simulink model "DS_distrIntp_1_10_simulated axes"  (R2019a)
settings: Solver=FixedStepDiscrete  StartTime=0.0  StopTime=inf  FixedStep=Ts  RelTol=1e-3
InitFcn:
  | %% Verwende vordefinierte Setpoints (Kreis mit Z-Komponente)
  | 
  | % Config
  | numCircles = 3;
  | scale=6;
  | %Versuch symmetrische Setpunkte zu setzen
  | pointsPerCircle =scale*(4+3*numCircles)+2;
  | 
  | r = 50;
  | m_x = r;
  | m_y = r;
  | 
  | % //
  | s = linspace(0,2*pi,pointsPerCircle);
  | 
  | setPoints_x = [];
  | setPoints_y = [];
  | 
  | for ii=1:numCircles
  | 
  | setPoints_x = [setPoints_x (-cos(s(1:floor(pointsPerCircle / 2))).*r + m_x + 2*r*(ii-1))]; %#ok<AGROW>
  | setPoints_y = [setPoints_y (sin(s).*r+m_y)]; %#ok<AGROW>pointsPerCircle / 2
  | 
  | end
  | 
  | setPoints_x = [setPoints_x flip(setPoints_x(1:end))];
  | 
  | % Loeschen doppelter y-Werte (Kreisuebergang)
  | setPoints_x(pointsPerCircle .* [1:numCircles]) = [];
  | setPoints_y(pointsPerCircle .* [1:numCircles]) = [];
  | 
  | % setPoints_x= [linspace(0,setPoints_x(19),19) setPoints_x(20:end)];
  | % setPoints_y= [linspace(0,setPoints_y(19),19) setPoints_y(20:end)];
  | 
  | % Array Elemente verschieben
  | % setPoints_x = circshift(setPoints_x,-pointsPerCircle/4,2);
  | % setPoints_y = circshift(setPoints_y,-pointsPerCircle/4,2);
  | 
  | z = zeros(1,size(setPoints_x,2));
  | z_x = -5:5;
  | z_y = -z_x.^2 + 25;
  | z_idx = 90;
  | z_idx2 = 210;
  | z(z_idx:z_idx+length(z_x)-1) = z_y;
  | z(z_idx2:z_idx2+length(z_x)-1) = z_y;
  | % z = [z_y z];
  | setPoints_z = z;
  | 
  | % setPoints_x = [zeros(1,length(z_y)) setPoints_x];
  | % setPoints_y = [setPoints_y(1,1)*ones(1,length(z_y)) setPoints_y];
  | 
  | % Umrechnung der Einheiten für Demonstrator
  | % setPoints_x = setPoints_x ./ 1000;
  | % setPoints_y = setPoints_y ./ 1000;
  | % setPoints_z = setPoints_z ./ 1000;
  | 
  | 
  | %{
  | plot(setPoints_x,setPoints_y);
  | fig = figure;
  | ... (+13 lines)
StartFcn:
  | close all;
model workspace (MAT data in the model file):
  MCOS : class17 (value not decoded)
  MCOS : class17 (value not decoded)
  MCOS : class17 (value not decoded)
  MCOS : class17 (value not decoded)
  MCOS : class17 (value not decoded)
  MCOS : class17 (value not decoded)
  MCOS : class17 (value not decoded)
  MCOS : class17 (value not decoded)
  MCOS : class17 (value not decoded)
  MCOS : class17 (value not decoded)
  MCOS : class17 (value not decoded)
  MCOS : class17 (value not decoded)
  MCOS : class17 (value not decoded)
  MCOS : class17 (value not decoded)
undefined symbols (not defined in the file or in its folder): DiscIntNeverNeededParam, VelOverride
libraries: simulink x19, vrlib x5, sldrtlib x2
(part 3 of 4)

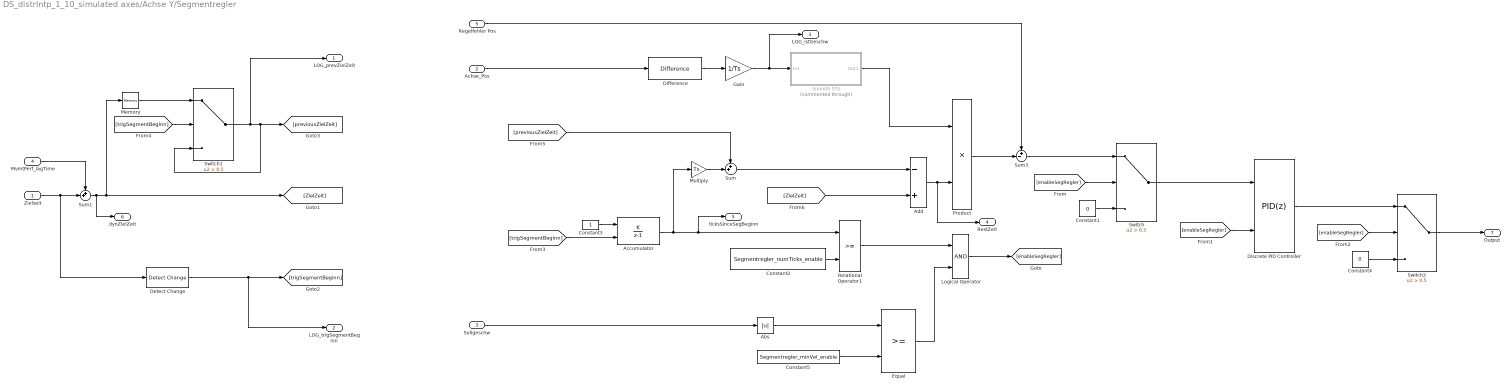
== system DS_distrIntp_1_10_simulated axes/Achse Y/Segmentregler ==
  Zielzeit : Inport
  Achse_Pos : Inport  Port=2
  Sollgeschw : Inport  Port=3
  MvmtPerf_lagTime : Inport  Port=4
  Regelfehler Pos : Inport  Port=5
  Abs : Abs
  Accumulator : DiscreteIntegrator  IntegratorMethod=Accumulation: Forward Euler  gainval=1  ExternalReset=rising  SampleTime=-1  ICPrevOutput=DiscIntNeverNeededParam  ICPrevScaledInput=DiscIntNeverNeededParam
  Add : Sum  Inputs=-+
  Constant1 : Constant  Value=0
  Constant2 : Constant  Value=Segmentregler_numTicks_enable
  Constant3 : Constant
  Constant4 : Constant  Value=0
  Constant5 : Constant  Value=Segmentregler_minVel_enable
  Detect Change : simulink/Logic and Bit Operations/Detect Change  vinit=0  OutDataTypeStr=boolean
  Difference : simulink/Discrete/Difference  ICPrevInput=0.0  OutMin=[]  OutMax=[]  OutDataType=fixdt(1, 16)  OutScaling=2^-10  DoSatur=off
  Discrete PID Controller : simulink/Continuous/PID Controller  Controller=PID  Form=Parallel  TimeDomain=Discrete-time  SampleTime=-1  IntegratorMethod=Forward Euler  FilterMethod=Forward Euler  ControllerParametersSource=internal  P=Segmentregler_P_Gain  I=Segmentregler_I_Gain  D=0  UseFilter=on  N=100  TunerSelectOption=Transfer Function Based (PID Tuner App)  InitialConditionSource=internal  InitialConditionForIntegrator=0  InitialConditionForFilter=0  DifferentiatorICPrevScaledInput=0  ExternalReset=falling  TrackingMode=off  Kt=1  LimitOutput=off  UpperSaturationLimit=inf  LowerSaturationLimit=-inf  LinearizeAsGain=off  AntiWindupMode=none  Kb=1  POutMin=[]  POutMax=[]  IOutMin=[]  IOutMax=[]  DOutMin=[]  DOutMax=[]  NOutMin=[]  NOutMax=[]  SumOutMin=[]  SumOutMax=[]  SaturationOutMin=[]  SaturationOutMax=[]  PParamMin=[]  PParamMax=[]  IParamMin=[]  IParamMax=[]  DParamMin=[]  DParamMax=[]  NParamMin=[]  NParamMax=[]  KbParamMin=[]  KbParamMax=[]  KtParamMin=[]  KtParamMax=[]  KbOutMin=[]  KbOutMax=[]  KtOutMin=[]  KtOutMax=[]  IntegratorOutMin=[]  IntegratorOutMax=[]  FilterOutMin=[]  FilterOutMax=[]  SumI1OutMin=[]  SumI1OutMax=[]  SumI2OutMin=[]  SumI2OutMax=[]  SumI3OutMin=[]  SumI3OutMax=[]  SumI4OutMin=[]  SumI4OutMax=[]  SumDOutMin=[]  SumDOutMax=[]  DifferentiatorOutMin=[]  DifferentiatorOutMax=[]  FilterDiffOutCoefMin=[]  FilterDiffOutCoefMax=[]  ReciprocalOutMin=[]  ReciprocalOutMax=[]  SumDenOutMin=[]  SumDenOutMax=[]  SumNumOutMin=[]  SumNumOutMax=[]  DivideOutMin=[]  DivideOutMax=[]  IntegratorContinuousStateAttributes=''  IntegratorStateMustResolveToSignalObject=off  IntegratorRTWStateStorageClass=Auto  FilterContinuousStateAttributes=''  FilterStateMustResolveToSignalObject=off  FilterRTWStateStorageClass=Auto  ParallelPVariant=InternalParameters  IdealPVariant=Disabled  IVariant=InternalParameters  DVariant=InternalParameters  IntegratorVariant=Discrete  SatVariant=Disabled  AWVariant=Passthrough  PCopyVariant=Disabled  TRVariant=Disabled  FdbkBlocksVariant=Forward  IdealPFdbkVariant=Disabled  SatFdbkVariant=Disabled  DerivativeFilterVariant=ForwardEulerFilter  NVariant=InternalParameters  NCopyVariant=Disabled  FilterICVariant=InternalICsFilter  IntegratorICVariant=InternalICs  ExternalResetVariant=ExternalReset  TRSumVariant=Passthrough  SumFdbkVariant=Disabled  SumVariant=Sum_PID
  Equal : RelationalOperator  OutDataTypeStr=boolean  RndMeth=Simplest
  Gain : Gain  Gain=1/Ts
  Logical Operator : Logic  AllPortsSameDT=off  OutDataTypeStr=boolean
  Memory : Memory
  Multiply : Gain  Gain=Ts
  Product : Product
  Relational Operator1 : RelationalOperator  OutDataTypeStr=boolean  RndMeth=Simplest
  Smooth 5Ts : Subsystem  Commented=through
  Sum : Sum  Inputs=++|
  Sum1 : Sum  Inputs=++|
  Sum3 : Sum  Inputs=+-|
  Switch : Switch  Criteria=u2 > Threshold  Threshold=0.5
  Switch1 : Switch  Criteria=u2 > Threshold  Threshold=0.5
  Switch2 : Switch  Criteria=u2 > Threshold  Threshold=0.5
  LOG_prevZielZeit : Outport  VectorParamsAs1DForOutWhenUnconnected=off
  LOG_trigSegmentBeginn : Outport  Port=2  VectorParamsAs1DForOutWhenUnconnected=off
  LOG_istGeschw : Outport  Port=3  VectorParamsAs1DForOutWhenUnconnected=off
  RestZeit : Outport  Port=4  VectorParamsAs1DForOutWhenUnconnected=off
  ticksSinceSegBeginn : Outport  Port=5  VectorParamsAs1DForOutWhenUnconnected=off
  dynZielZeit : Outport  Port=6  VectorParamsAs1DForOutWhenUnconnected=off
  Output : Outport  Port=7  VectorParamsAs1DForOutWhenUnconnected=off
  wires:
  MvmtPerf_lagTime/1 -> Sum1/1
  Zielzeit/1 -> Sum1/2, Detect Change/1
  Abs/1 -> Equal/1
  Sum1/1 -> [ZielZeit], Memory/1, dynZielZeit/1
  [ZielZeit] -> Add/2
  Multiply/1 -> Sum/2
  Smooth 5Ts/1(Out1) -> Product/1
  [previousZielZeit] -> Sum/1
  Switch1/1 -> [previousZielZeit], Switch1/3, LOG_prevZielZeit/1
  [trigSegmentBeginn] -> Switch1/2
  [trigSegmentBeginn] -> Accumulator/2
  Detect Change/1 -> [trigSegmentBeginn], LOG_trigSegmentBeginn/1
  Gain/1 -> Smooth 5Ts/1(In1), LOG_istGeschw/1
  Memory/1 -> Switch1/1
  Equal/1 -> Logical Operator/2
  Constant5/1 -> Equal/2
  Sollgeschw/1 -> Abs/1
  [enableSegRegler] -> Switch2/2
  [enableSegRegler] -> Discrete PID Controller/2
  [enableSegRegler] -> Switch/2
  Logical Operator/1 -> [enableSegRegler]
  Switch2/1 -> Output/1
  Regelfehler Pos/1 -> Sum3/1
  Product/1 -> Sum3/2
  Constant4/1 -> Switch2/3
  Constant1/1 -> Switch/3
  Discrete PID Controller/1 -> Switch2/1
  Achse_Pos/1 -> Difference/1
  Constant2/1 -> Relational Operator1/2
  Add/1 -> Product/2, RestZeit/1
  Relational Operator1/1 -> Logical Operator/1
  Sum/1 -> Add/1
  Switch/1 -> Discrete PID Controller/1
  Sum3/1 -> Switch/1
  Difference/1 -> Gain/1
  Accumulator/1 -> Relational Operator1/1, ticksSinceSegBeginn/1, Multiply/1
  Constant3/1 -> Accumulator/1

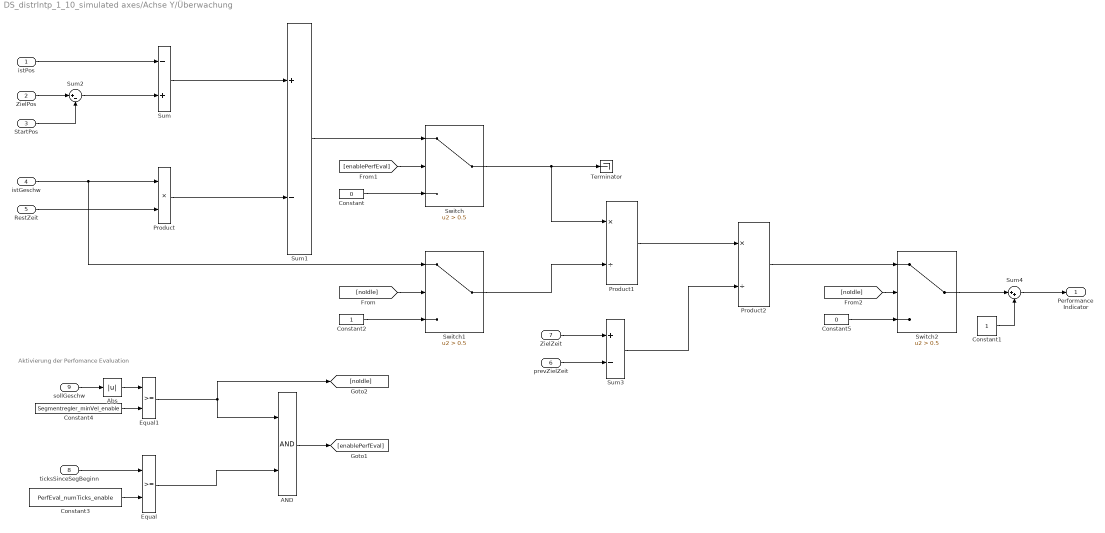
== system DS_distrIntp_1_10_simulated axes/Achse Y/Überwachung ==
  note: Aktivierung der Perfomance Evaluation
  istPos : Inport
  ZielPos : Inport  Port=2
  StartPos : Inport  Port=3
  istGeschw : Inport  Port=4
  RestZeit : Inport  Port=5
  prevZielZeit : Inport  Port=6
  ZielZeit : Inport  Port=7
  ticksSinceSegBeginn : Inport  Port=8
  sollGeschw : Inport  Port=9
  AND : Logic  AllPortsSameDT=off  OutDataTypeStr=boolean
  Abs : Abs
  Constant : Constant  Value=0
  Constant1 : Constant
  Constant2 : Constant
  Constant3 : Constant  Value=PerfEval_numTicks_enable
  Constant4 : Constant  Value=Segmentregler_minVel_enable
  Constant5 : Constant  Value=0
  Equal : RelationalOperator  OutDataTypeStr=boolean  RndMeth=Simplest
  Equal1 : RelationalOperator  OutDataTypeStr=boolean  RndMeth=Simplest
  Product : Product
  Product1 : Product  Inputs=*/
  Product2 : Product  Inputs=*/
  Sum : Sum  Inputs=-+
  Sum1 : Sum  Inputs=+-
  Sum2 : Sum  Inputs=|+-
  Sum3 : Sum  Inputs=+-
  Sum4 : Sum  Inputs=|++
  Switch : Switch  Criteria=u2 > Threshold  Threshold=0.5
  Switch1 : Switch  Criteria=u2 > Threshold  Threshold=0.5
  Switch2 : Switch  Criteria=u2 > Threshold  Threshold=0.5
  Terminator : Terminator
  Performance Indicator : Outport  VectorParamsAs1DForOutWhenUnconnected=off
  wires:
  Abs/1 -> Equal1/1
  Constant5/1 -> Switch2/3
  [noIdle] -> Switch2/2
  Product2/1 -> Switch2/1
  Switch2/1 -> Sum4/1
  Switch1/1 -> Product1/2
  Constant2/1 -> Switch1/3
  [noIdle] -> Switch1/2
  AND/1 -> [enablePerfEval]
  Equal1/1 -> AND/1, [noIdle]
  Constant4/1 -> Equal1/2
  sollGeschw/1 -> Abs/1
  Equal/1 -> AND/2
  Constant3/1 -> Equal/2
  ticksSinceSegBeginn/1 -> Equal/1
  Constant1/1 -> Sum4/2
  Sum4/1 -> Performance Indicator/1
  ZielZeit/1 -> Sum3/1
  prevZielZeit/1 -> Sum3/2
  Sum3/1 -> Product2/2
  Product1/1 -> Product2/1
  Constant/1 -> Switch/3
  [enablePerfEval] -> Switch/2
  Switch/1 -> Terminator/1, Product1/1
  Sum1/1 -> Switch/1
  Sum2/1 -> Sum/2
  StartPos/1 -> Sum2/2
  ZielPos/1 -> Sum2/1
  Sum/1 -> Sum1/1
  Product/1 -> Sum1/2
  RestZeit/1 -> Product/2
  istGeschw/1 -> Product/1, Switch1/1
  istPos/1 -> Sum/1

== system DS_distrIntp_1_10_simulated axes/Achse Z/Sat_maxGeschw ==
  Threshold : Inport
  In : Inport  Port=2
  Abs : Abs
  Multiply : Gain  Gain=-1
  Sign : Signum
  Sum3 : Sum  Inputs=-+
  Switch : Switch  Criteria=u2 > Threshold
  Switch1 : Switch
  Out : Outport  VectorParamsAs1DForOutWhenUnconnected=off
  wires:
  Switch1/1 -> Out/1
  Multiply/1 -> Switch1/3
  Switch/1 -> Switch1/1, Multiply/1
  Sign/1 -> Switch1/2
  In/1 -> Abs/1, Sign/1
  Abs/1 -> Switch/3, Sum3/2
  Threshold/1 -> Sum3/1, Switch/1
  Sum3/1 -> Switch/2

== system DS_distrIntp_1_10_simulated axes/Achse Z/Sat_sollGeschw ==
  Threshold : Inport
  In : Inport  Port=2
  Abs : Abs
  Constant : Constant  Value=minAllowedVelSaturation
  Max : MinMax  Function=max  Inputs=2
  Multiply : Gain  Gain=-1
  Sign : Signum
  Sum3 : Sum  Inputs=-+
  Switch : Switch  Criteria=u2 > Threshold
  Switch1 : Switch
  Out : Outport  VectorParamsAs1DForOutWhenUnconnected=off
  wires:
  Sum3/1 -> Switch/2
  Max/1 -> Switch/1, Sum3/1
  Abs/1 -> Sum3/2, Switch/3
  In/1 -> Sign/1, Abs/1
  Sign/1 -> Switch1/2
  Switch/1 -> Multiply/1, Switch1/1
  Multiply/1 -> Switch1/3
  Switch1/1 -> Out/1
  Threshold/1 -> Max/1
  Constant/1 -> Max/2

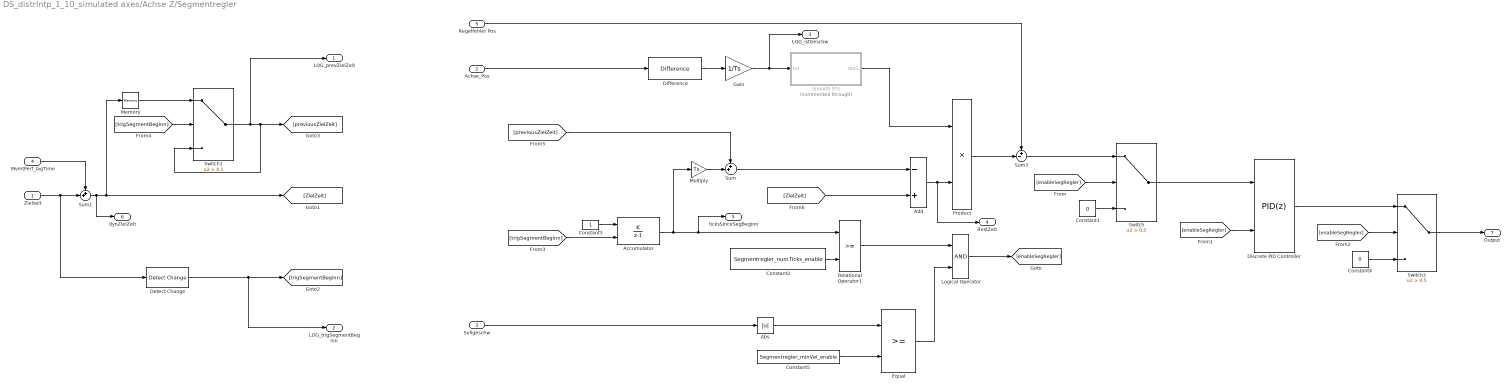
== system DS_distrIntp_1_10_simulated axes/Achse Z/Segmentregler ==
  Zielzeit : Inport
  Achse_Pos : Inport  Port=2
  Sollgeschw : Inport  Port=3
  MvmtPerf_lagTime : Inport  Port=4
  Regelfehler Pos : Inport  Port=5
  Abs : Abs
  Accumulator : DiscreteIntegrator  IntegratorMethod=Accumulation: Forward Euler  gainval=1  ExternalReset=rising  SampleTime=-1  ICPrevOutput=DiscIntNeverNeededParam  ICPrevScaledInput=DiscIntNeverNeededParam
  Add : Sum  Inputs=-+
  Constant1 : Constant  Value=0
  Constant2 : Constant  Value=Segmentregler_numTicks_enable
  Constant3 : Constant
  Constant4 : Constant  Value=0
  Constant5 : Constant  Value=Segmentregler_minVel_enable
  Detect Change : simulink/Logic and Bit Operations/Detect Change  vinit=0  OutDataTypeStr=boolean
  Difference : simulink/Discrete/Difference  ICPrevInput=0.0  OutMin=[]  OutMax=[]  OutDataType=fixdt(1, 16)  OutScaling=2^-10  DoSatur=off
  Discrete PID Controller : simulink/Continuous/PID Controller  Controller=PID  Form=Parallel  TimeDomain=Discrete-time  SampleTime=-1  IntegratorMethod=Forward Euler  FilterMethod=Forward Euler  ControllerParametersSource=internal  P=Segmentregler_P_Gain  I=Segmentregler_I_Gain  D=0  UseFilter=on  N=100  TunerSelectOption=Transfer Function Based (PID Tuner App)  InitialConditionSource=internal  InitialConditionForIntegrator=0  InitialConditionForFilter=0  DifferentiatorICPrevScaledInput=0  ExternalReset=falling  TrackingMode=off  Kt=1  LimitOutput=off  UpperSaturationLimit=inf  LowerSaturationLimit=-inf  LinearizeAsGain=off  AntiWindupMode=none  Kb=1  POutMin=[]  POutMax=[]  IOutMin=[]  IOutMax=[]  DOutMin=[]  DOutMax=[]  NOutMin=[]  NOutMax=[]  SumOutMin=[]  SumOutMax=[]  SaturationOutMin=[]  SaturationOutMax=[]  PParamMin=[]  PParamMax=[]  IParamMin=[]  IParamMax=[]  DParamMin=[]  DParamMax=[]  NParamMin=[]  NParamMax=[]  KbParamMin=[]  KbParamMax=[]  KtParamMin=[]  KtParamMax=[]  KbOutMin=[]  KbOutMax=[]  KtOutMin=[]  KtOutMax=[]  IntegratorOutMin=[]  IntegratorOutMax=[]  FilterOutMin=[]  FilterOutMax=[]  SumI1OutMin=[]  SumI1OutMax=[]  SumI2OutMin=[]  SumI2OutMax=[]  SumI3OutMin=[]  SumI3OutMax=[]  SumI4OutMin=[]  SumI4OutMax=[]  SumDOutMin=[]  SumDOutMax=[]  DifferentiatorOutMin=[]  DifferentiatorOutMax=[]  FilterDiffOutCoefMin=[]  FilterDiffOutCoefMax=[]  ReciprocalOutMin=[]  ReciprocalOutMax=[]  SumDenOutMin=[]  SumDenOutMax=[]  SumNumOutMin=[]  SumNumOutMax=[]  DivideOutMin=[]  DivideOutMax=[]  IntegratorContinuousStateAttributes=''  IntegratorStateMustResolveToSignalObject=off  IntegratorRTWStateStorageClass=Auto  FilterContinuousStateAttributes=''  FilterStateMustResolveToSignalObject=off  FilterRTWStateStorageClass=Auto  ParallelPVariant=InternalParameters  IdealPVariant=Disabled  IVariant=InternalParameters  DVariant=InternalParameters  IntegratorVariant=Discrete  SatVariant=Disabled  AWVariant=Passthrough  PCopyVariant=Disabled  TRVariant=Disabled  FdbkBlocksVariant=Forward  IdealPFdbkVariant=Disabled  SatFdbkVariant=Disabled  DerivativeFilterVariant=ForwardEulerFilter  NVariant=InternalParameters  NCopyVariant=Disabled  FilterICVariant=InternalICsFilter  IntegratorICVariant=InternalICs  ExternalResetVariant=ExternalReset  TRSumVariant=Passthrough  SumFdbkVariant=Disabled  SumVariant=Sum_PID
  Equal : RelationalOperator  OutDataTypeStr=boolean  RndMeth=Simplest
  Gain : Gain  Gain=1/Ts
  Logical Operator : Logic  AllPortsSameDT=off  OutDataTypeStr=boolean
  Memory : Memory
  Multiply : Gain  Gain=Ts
  Product : Product
  Relational Operator1 : RelationalOperator  OutDataTypeStr=boolean  RndMeth=Simplest
  Smooth 5Ts : Subsystem  Commented=through
  Sum : Sum  Inputs=++|
  Sum1 : Sum  Inputs=++|
  Sum3 : Sum  Inputs=+-|
  Switch : Switch  Criteria=u2 > Threshold  Threshold=0.5
  Switch1 : Switch  Criteria=u2 > Threshold  Threshold=0.5
  Switch2 : Switch  Criteria=u2 > Threshold  Threshold=0.5
  LOG_prevZielZeit : Outport  VectorParamsAs1DForOutWhenUnconnected=off
  LOG_trigSegmentBeginn : Outport  Port=2  VectorParamsAs1DForOutWhenUnconnected=off
  LOG_istGeschw : Outport  Port=3  VectorParamsAs1DForOutWhenUnconnected=off
  RestZeit : Outport  Port=4  VectorParamsAs1DForOutWhenUnconnected=off
  ticksSinceSegBeginn : Outport  Port=5  VectorParamsAs1DForOutWhenUnconnected=off
  dynZielZeit : Outport  Port=6  VectorParamsAs1DForOutWhenUnconnected=off
  Output : Outport  Port=7  VectorParamsAs1DForOutWhenUnconnected=off
  wires:
  Constant3/1 -> Accumulator/1
  Accumulator/1 -> Multiply/1, ticksSinceSegBeginn/1, Relational Operator1/1
  Difference/1 -> Gain/1
  Sum3/1 -> Switch/1
  Switch/1 -> Discrete PID Controller/1
  Sum/1 -> Add/1
  Relational Operator1/1 -> Logical Operator/1
  Add/1 -> RestZeit/1, Product/2
  Constant2/1 -> Relational Operator1/2
  Achse_Pos/1 -> Difference/1
  Discrete PID Controller/1 -> Switch2/1
  Constant1/1 -> Switch/3
  Constant4/1 -> Switch2/3
  Product/1 -> Sum3/2
  Regelfehler Pos/1 -> Sum3/1
  Switch2/1 -> Output/1
  Logical Operator/1 -> [enableSegRegler]
  [enableSegRegler] -> Switch/2
  [enableSegRegler] -> Discrete PID Controller/2
  [enableSegRegler] -> Switch2/2
  Sollgeschw/1 -> Abs/1
  Constant5/1 -> Equal/2
  Equal/1 -> Logical Operator/2
  Memory/1 -> Switch1/1
  Gain/1 -> LOG_istGeschw/1, Smooth 5Ts/1(In1)
  Detect Change/1 -> LOG_trigSegmentBeginn/1, [trigSegmentBeginn]
  [trigSegmentBeginn] -> Accumulator/2
  [trigSegmentBeginn] -> Switch1/2
  Switch1/1 -> LOG_prevZielZeit/1, Switch1/3, [previousZielZeit]
  [previousZielZeit] -> Sum/1
  Smooth 5Ts/1(Out1) -> Product/1
  Multiply/1 -> Sum/2
  [ZielZeit] -> Add/2
  Sum1/1 -> dynZielZeit/1, Memory/1, [ZielZeit]
  Abs/1 -> Equal/1
  Zielzeit/1 -> Detect Change/1, Sum1/2
  MvmtPerf_lagTime/1 -> Sum1/1

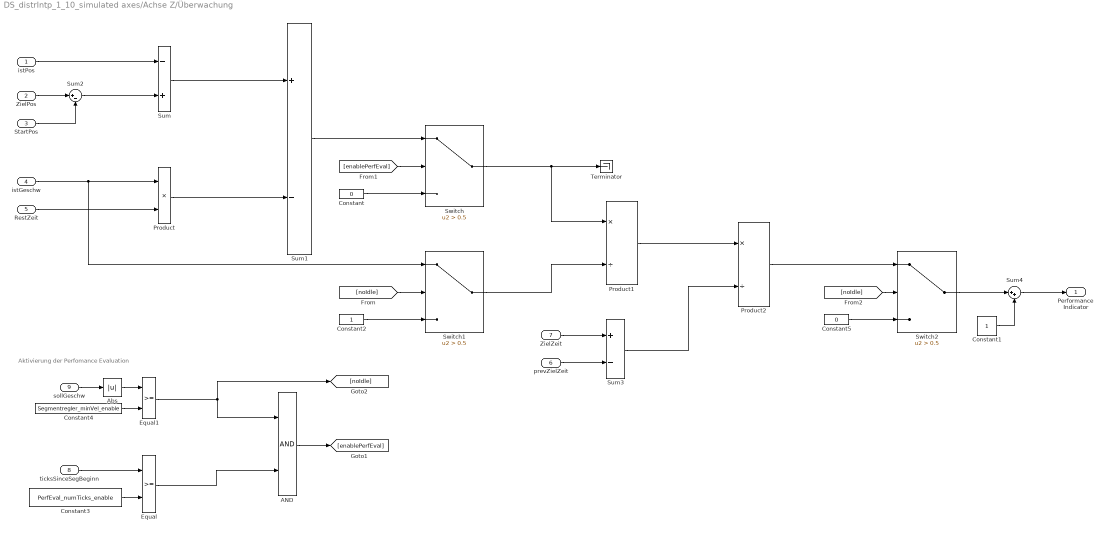
== system DS_distrIntp_1_10_simulated axes/Achse Z/Überwachung ==
  note: Aktivierung der Perfomance Evaluation
  istPos : Inport
  ZielPos : Inport  Port=2
  StartPos : Inport  Port=3
  istGeschw : Inport  Port=4
  RestZeit : Inport  Port=5
  prevZielZeit : Inport  Port=6
  ZielZeit : Inport  Port=7
  ticksSinceSegBeginn : Inport  Port=8
  sollGeschw : Inport  Port=9
  AND : Logic  AllPortsSameDT=off  OutDataTypeStr=boolean
  Abs : Abs
  Constant : Constant  Value=0
  Constant1 : Constant
  Constant2 : Constant
  Constant3 : Constant  Value=PerfEval_numTicks_enable
  Constant4 : Constant  Value=Segmentregler_minVel_enable
  Constant5 : Constant  Value=0
  Equal : RelationalOperator  OutDataTypeStr=boolean  RndMeth=Simplest
  Equal1 : RelationalOperator  OutDataTypeStr=boolean  RndMeth=Simplest
  Product : Product
  Product1 : Product  Inputs=*/
  Product2 : Product  Inputs=*/
  Sum : Sum  Inputs=-+
  Sum1 : Sum  Inputs=+-
  Sum2 : Sum  Inputs=|+-
  Sum3 : Sum  Inputs=+-
  Sum4 : Sum  Inputs=|++
  Switch : Switch  Criteria=u2 > Threshold  Threshold=0.5
  Switch1 : Switch  Criteria=u2 > Threshold  Threshold=0.5
  Switch2 : Switch  Criteria=u2 > Threshold  Threshold=0.5
  Terminator : Terminator
  Performance Indicator : Outport  VectorParamsAs1DForOutWhenUnconnected=off
  wires:
  istPos/1 -> Sum/1
  istGeschw/1 -> Switch1/1, Product/1
  RestZeit/1 -> Product/2
  Product/1 -> Sum1/2
  Sum/1 -> Sum1/1
  ZielPos/1 -> Sum2/1
  StartPos/1 -> Sum2/2
  Sum2/1 -> Sum/2
  Sum1/1 -> Switch/1
  Switch/1 -> Product1/1, Terminator/1
  [enablePerfEval] -> Switch/2
  Constant/1 -> Switch/3
  Product1/1 -> Product2/1
  Sum3/1 -> Product2/2
  prevZielZeit/1 -> Sum3/2
  ZielZeit/1 -> Sum3/1
  Sum4/1 -> Performance Indicator/1
  Constant1/1 -> Sum4/2
  ticksSinceSegBeginn/1 -> Equal/1
  Constant3/1 -> Equal/2
  Equal/1 -> AND/2
  sollGeschw/1 -> Abs/1
  Constant4/1 -> Equal1/2
  Equal1/1 -> [noIdle], AND/1
  AND/1 -> [enablePerfEval]
  [noIdle] -> Switch1/2
  Constant2/1 -> Switch1/3
  Switch1/1 -> Product1/2
  Switch2/1 -> Sum4/1
  Product2/1 -> Switch2/1
  [noIdle] -> Switch2/2
  Constant5/1 -> Switch2/3
  Abs/1 -> Equal1/1

== system DS_distrIntp_1_10_simulated axes/Joystick Ctrl/Fetch_Global_Data ==
  Chart : Stateflow chart  BlockKeywords=__PRM__SERIALIZED__DATA__:Stateflow Chart,Stateflow Diagram  TreatAsAtomicUnit=on  SystemSampleTime=0.2
  Mux : Mux  Inputs=6
  Terminator : Terminator
  wires:
  Chart/2(velOR_y) -> Mux/2
  Chart/1(velOR_x) -> Mux/1
  Chart/6(vel_z) -> Mux/6
  Chart/4(vel_x) -> Mux/4
  Chart/5(vel_y) -> Mux/5
  Chart/3(velOR_z) -> Mux/3
  Mux/1 -> Terminator/1

== system DS_distrIntp_1_10_simulated axes/Joystick Ctrl/Joystick ==
  AchseX : Subsystem
  AchseY : Subsystem
  AchseZ : Subsystem
  Bus Creator : BusCreator  Inputs=2
  Joystick Input : vrlib/Joystick Input  joyid=1  adjustports=off  forcefeed=off
      settings: SourceProductName=Simulink
  wires:
  Joystick Input/2 -> Bus Creator/2
  Joystick Input/1 -> Bus Creator/1
  Bus Creator/1 -> AchseZ/1(Inport), AchseX/1(Inport), AchseY/1(Inport)

== system DS_distrIntp_1_10_simulated axes/Joystick Ctrl/Sliders ==
  Constant : Constant  Value=0.1294117647058824
  Constant1 : Constant  Value=0.1529411764705882
  Constant2 : Constant  Value=0.1058823529411765
  Constant3 : Constant  Value=0.125
  Constant4 : Constant  Value=0.125
  Constant5 : Constant  Value=0.125
  Data Store Write : DataStoreWrite  DataStoreName=VelOverride  SampleTime=0.5  DataStoreElements=VelOverride(1)
  Data Store Write1 : DataStoreWrite  DataStoreName=VelOverride  SampleTime=0.5  DataStoreElements=VelOverride(2)
  Data Store Write2 : DataStoreWrite  DataStoreName=VelOverride  SampleTime=0.5  DataStoreElements=VelOverride(3)
  Min : MinMax  Function=max  Inputs=2
  Min1 : MinMax  Function=max  Inputs=2
  Min2 : MinMax  Function=max  Inputs=2
  wires:
  Constant3/1 -> Min/1
  Constant/1 -> Min/2
  Min/1 -> Data Store Write/1
  Constant4/1 -> Min1/1
  Constant1/1 -> Min1/2
  Min1/1 -> Data Store Write1/1
  Constant5/1 -> Min2/1
  Constant2/1 -> Min2/2
  Min2/1 -> Data Store Write2/1

== system DS_distrIntp_1_10_simulated axes/Achse X/Segmentregler/Smooth 5Ts ==
  In1 : Inport
  Delay{,1..3} (4 alike) : Delay  DelayLength=1
  Gain : Gain  Gain=1/5
  Sum : Sum  Inputs=+++++
  Out1 : Outport  VectorParamsAs1DForOutWhenUnconnected=off
  wires:
  In1/1 -> Sum/5, Delay/1
  Delay/1 -> Sum/4, Delay1/1
  Delay1/1 -> Sum/3, Delay2/1
  Delay2/1 -> Sum/2, Delay3/1
  Delay3/1 -> Sum/1
  Sum/1 -> Gain/1
  Gain/1 -> Out1/1

== system DS_distrIntp_1_10_simulated axes/Achse Y/Segmentregler/Smooth 5Ts ==
  In1 : Inport
  Delay{,1..3} (4 alike) : Delay  DelayLength=1
  Gain : Gain  Gain=1/5
  Sum : Sum  Inputs=+++++
  Out1 : Outport  VectorParamsAs1DForOutWhenUnconnected=off
  wires:
  Gain/1 -> Out1/1
  Sum/1 -> Gain/1
  Delay3/1 -> Sum/1
  Delay2/1 -> Delay3/1, Sum/2
  Delay1/1 -> Delay2/1, Sum/3
  Delay/1 -> Delay1/1, Sum/4
  In1/1 -> Delay/1, Sum/5

== system DS_distrIntp_1_10_simulated axes/Achse Z/Segmentregler/Smooth 5Ts ==
  In1 : Inport
  Delay{,1..3} (4 alike) : Delay  DelayLength=1
  Gain : Gain  Gain=1/5
  Sum : Sum  Inputs=+++++
  Out1 : Outport  VectorParamsAs1DForOutWhenUnconnected=off
  wires:
  In1/1 -> Sum/5, Delay/1
  Delay/1 -> Sum/4, Delay1/1
  Delay1/1 -> Sum/3, Delay2/1
  Delay2/1 -> Sum/2, Delay3/1
  Delay3/1 -> Sum/1
  Sum/1 -> Gain/1
  Gain/1 -> Out1/1

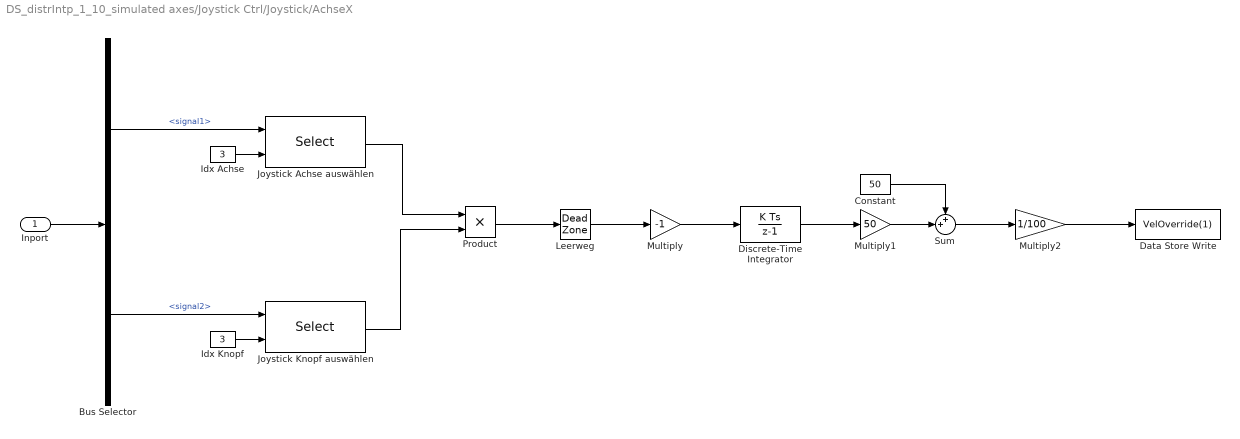
== system DS_distrIntp_1_10_simulated axes/Joystick Ctrl/Joystick/AchseX ==
  Inport : Inport
  Bus Selector : BusSelector  OutputSignals=signal1,signal2
  Constant : Constant  Value=50
  Data Store Write : DataStoreWrite  DataStoreName=VelOverride  SampleTime=0.5  DataStoreElements=VelOverride(1)
  Discrete-Time Integrator : DiscreteIntegrator  gainval=0.5  SampleTime=-1  LimitOutput=on  UpperSaturationLimit=1  LowerSaturationLimit=-0.75  ICPrevOutput=DiscIntNeverNeededParam  ICPrevScaledInput=DiscIntNeverNeededParam
  Idx Achse : Constant  Value=3
  Idx Knopf : Constant  Value=3
  Joystick Achse auswählen : Selector  InputPortWidth=8  IndexOptions=Index vector (port)  Indices=[3]  OutputSizes=1
  Joystick Knopf auswählen : Selector  InputPortWidth=32  IndexOptions=Index vector (port)  Indices=[3]  OutputSizes=1
  Leerweg : DeadZone  LowerValue=-0.3  UpperValue=0.3  SaturateOnIntegerOverflow=on
  Multiply : Gain  Gain=-1
  Multiply1 : Gain  Gain=50
  Multiply2 : Gain  Gain=1/100
  Product : Product
  Sum : Sum  Inputs=++|
  wires:
  Multiply1/1 -> Sum/2
  Multiply/1 -> Discrete-Time Integrator/1
  Discrete-Time Integrator/1 -> Multiply1/1
  Constant/1 -> Sum/1
  Leerweg/1 -> Multiply/1
  Joystick Achse auswählen/1 -> Product/1
  Joystick Knopf auswählen/1 -> Product/2
  Product/1 -> Leerweg/1
  Sum/1 -> Multiply2/1
  Multiply2/1 -> Data Store Write/1
  Idx Achse/1 -> Joystick Achse auswählen/2
  Idx Knopf/1 -> Joystick Knopf auswählen/2
  Bus Selector/1 -> Joystick Achse auswählen/1  "<signal1>"
  Bus Selector/2 -> Joystick Knopf auswählen/1  "<signal2>"
  Inport/1 -> Bus Selector/1

== system DS_distrIntp_1_10_simulated axes/Joystick Ctrl/Joystick/AchseY ==
  Inport : Inport
  Bus Selector : BusSelector  OutputSignals=signal1,signal2
  Constant : Constant  Value=50
  Data Store Write : DataStoreWrite  DataStoreName=VelOverride  SampleTime=0.5  DataStoreElements=VelOverride(2)
  Discrete-Time Integrator : DiscreteIntegrator  gainval=0.5  SampleTime=-1  LimitOutput=on  UpperSaturationLimit=1  LowerSaturationLimit=-0.75  ICPrevOutput=DiscIntNeverNeededParam  ICPrevScaledInput=DiscIntNeverNeededParam
  Idx Achse : Constant  Value=3
  Idx Knopf : Constant  Value=4
  Joystick Achse auswählen : Selector  InputPortWidth=8  IndexOptions=Index vector (port)  Indices=[3]  OutputSizes=1
  Joystick Knopf auswählen : Selector  InputPortWidth=32  IndexOptions=Index vector (port)  Indices=[3]  OutputSizes=1
  Leerweg : DeadZone  LowerValue=-0.3  UpperValue=0.3  SaturateOnIntegerOverflow=on
  Multiply : Gain  Gain=-1
  Multiply1 : Gain  Gain=50
  Multiply2 : Gain  Gain=1/100
  Product : Product
  Sum : Sum  Inputs=++|
  wires:
  Inport/1 -> Bus Selector/1
  Bus Selector/2 -> Joystick Knopf auswählen/1  "<signal2>"
  Bus Selector/1 -> Joystick Achse auswählen/1  "<signal1>"
  Idx Knopf/1 -> Joystick Knopf auswählen/2
  Idx Achse/1 -> Joystick Achse auswählen/2
  Multiply2/1 -> Data Store Write/1
  Sum/1 -> Multiply2/1
  Product/1 -> Leerweg/1
  Joystick Knopf auswählen/1 -> Product/2
  Joystick Achse auswählen/1 -> Product/1
  Leerweg/1 -> Multiply/1
  Constant/1 -> Sum/1
  Discrete-Time Integrator/1 -> Multiply1/1
  Multiply/1 -> Discrete-Time Integrator/1
  Multiply1/1 -> Sum/2

== system DS_distrIntp_1_10_simulated axes/Joystick Ctrl/Joystick/AchseZ ==
  Inport : Inport
  Bus Selector : BusSelector  OutputSignals=signal1,signal2
  Constant : Constant  Value=50
  Data Store Write : DataStoreWrite  DataStoreName=VelOverride  SampleTime=0.5  DataStoreElements=VelOverride(3)
  Discrete-Time Integrator : DiscreteIntegrator  gainval=0.5  SampleTime=-1  LimitOutput=on  UpperSaturationLimit=1  LowerSaturationLimit=-0.75  ICPrevOutput=DiscIntNeverNeededParam  ICPrevScaledInput=DiscIntNeverNeededParam
  Idx Achse : Constant  Value=3
  Idx Knopf : Constant
  Joystick Achse auswählen : Selector  InputPortWidth=8  IndexOptions=Index vector (port)  Indices=[3]  OutputSizes=1
  Joystick Knopf auswählen : Selector  InputPortWidth=32  IndexOptions=Index vector (port)  Indices=[3]  OutputSizes=1
  Leerweg : DeadZone  LowerValue=-0.3  UpperValue=0.3  SaturateOnIntegerOverflow=on
  Multiply : Gain  Gain=-1
  Multiply1 : Gain  Gain=50
  Multiply2 : Gain  Gain=1/100
  Product : Product
  Sum : Sum  Inputs=++|
  wires:
  Multiply1/1 -> Sum/2
  Multiply/1 -> Discrete-Time Integrator/1
  Discrete-Time Integrator/1 -> Multiply1/1
  Constant/1 -> Sum/1
  Leerweg/1 -> Multiply/1
  Joystick Achse auswählen/1 -> Product/1
  Joystick Knopf auswählen/1 -> Product/2
  Product/1 -> Leerweg/1
  Sum/1 -> Multiply2/1
  Multiply2/1 -> Data Store Write/1
  Idx Achse/1 -> Joystick Achse auswählen/2
  Idx Knopf/1 -> Joystick Knopf auswählen/2
  Bus Selector/1 -> Joystick Achse auswählen/1  "<signal1>"
  Bus Selector/2 -> Joystick Knopf auswählen/1  "<signal2>"
  Inport/1 -> Bus Selector/1

== stateflow chart DS_distrIntp_1_10_simulated axes/MASTER ==
  state funcs [group]
  state Dispatcher [parallel]
    settings: executionOrder=1
    state Idle
    state Registriere_Achse
      entry: num_registeredAxes = ...
      num_registeredAxes + 1;
    state Erhalte_Koordinationsvektor
      entry:
      num_collectedCVectors = ...
      num_collectedCVectors + 1;
      cVectors = [cVectors; cVector_exchange];
      FLAG_canSend_cVector = 1;
    state Distribute_Coordination_Info
      entry:
      FLAG_cVectors_complete = 1;
    state Registriere_Achsen_bereit
      entry:
      num_readyAxes = num_readyAxes + 1;
      if(num_readyAxes == num_registeredAxes)
      FLAG_allAxesReady = 1;
      end
    state DONE
      entry:
      num_doneAxes = num_doneAxes + 1;
      if num_doneAxes == num_registeredAxes
      FLAG_stopSim = 1;
      end
    state Movement_Performance_Evaluation
      entry:
      while receive(MvmtPerfCoeff)
      if MvmtPerfCoeff.data > MvmtPerf
      MvmtPerf = MvmtPerfCoeff.data;
      end
      if MvmtPerfCoeff.data == -1
      MvmtPerf = 1;
      end
      discard(MvmtPerfCoeff);
      end
    (default) -> Idle
    Idle -> Registriere_Achse [order 1] : registerAxis
    Registriere_Achse -> Idle
    Idle -> Erhalte_Koordinationsvektor [order 2] : cVector_sent
    Erhalte_Koordinationsvektor -> Idle
    Idle -> Distribute_Coordination_Info [order 3] : [num_collectedCVectors==...
        | num_registeredAxes && ...
        | FLAG_cVectors_complete == 0]
    Distribute_Coordination_Info -> Idle
    Idle -> Registriere_Achsen_bereit [order 4] : axis_ready
    Registriere_Achsen_bereit -> Idle
    Idle -> Dispatcher.DONE [order 5] : axis_done
    Dispatcher.DONE -> Idle
    Idle -> Movement_Performance_Evaluation [order 6] : MvmtPerfCoeff
    Movement_Performance_Evaluation -> Idle
  state Axis_X [parallel]
    settings: executionOrder=2
    state Start_Idle
      entry:
      registerAxis.data = true;
      send(registerAxis)
    state Hermite_Interpolation
      entry:
      if FLAG_doAkima == 1
      iP = funcs.DS_hermIntp(setP,setP_dist);
      else
      iP = setP;
      end
    state Koordinationsvektor
      entry:
      cVector_init = funcs.DS_gen_Cvector_init...
      (iP,PAR_isAxis,PAR_maxVel);
    state Koordinationsvektor_austauschen
      during:
      if FLAG_canSend_cVector == 1
      cVector_exchange = cVector_init;
      FLAG_canSend_cVector = 0;
      send(cVector_sent);
      axisHasSentCVector = 1;
      end
      Axis_X.Koordinationsvektor_austauschen -> Axis_X.Koordinationsvektor_austauschen [order 1]
    state Wait_for_cVectors
    state Find_Consensus
      entry: execVec = funcs.DS_find_Consensus(iP,cVectors,...
      PAR_execIteratorStepSize,PAR_isAxis);
      send(axis_ready);
    state Start_run
      entry:
      RUN_idx = 0;
      RUN_startPos(1,PAR_isAxis) = setP(PAR_isAxis,1);
      RUN_num_steps = size(execVec,2);
      state Send_command
        entry:
        RUN_idx = RUN_idx + 1;
        currCVector = cVectors(:,RUN_idx)' ./ VelOverride';
        currCVal = max(currCVector);
        currOverrideAdaptationFactor = execVec(3,RUN_idx) / currCVal; %individueller neuer Override Faktor für diese Achse
        currStepTimeLength = execVec(3,RUN_idx) / currOverrideAdaptationFactor;
        RUN_pos(1,PAR_isAxis) = execVec(1,RUN_idx);
        RUN_vel(1,PAR_isAxis) = execVec(2,RUN_idx) * currOverrideAdaptationFactor;
        MvmtPerf_accumulatedLagTime = MvmtPerf_accumulatedLagTime + (currStepTimeLength - execVec(3,RUN_idx));
        RUN_time(1,PAR_isAxis) = execVec(4,RUN_idx) + MvmtPerf_accumulatedLagTime; %wird nicht benutzt
        RUN_maxVel(1,PAR_isAxis) = PAR_maxVel;
        RUN_MvmtPerfFeedback(1,PAR_isAxis) = 0; %wird zZt nicht benutzt
      state execute_movement
        state idle
          entry:
          MvmtPerfCoeff.data = -1;
          send(MvmtPerfCoeff);
        state getOwnPerfCoeff [commented out]
          entry:
          MvmtPerfCoeff.data = GET_perfIndicator(PAR_isAxis);
          send(MvmtPerfCoeff);
        state getMutualPerformance [commented out]
          entry:
          MvmtPerf_accumulatedLagTime = MvmtPerf_accumulatedLagTime + (MvmtPerf-1) * currStepTimeLength;
          RUN_MvmtPerfFeedback(1,PAR_isAxis) = (MvmtPerf-1) * currStepTimeLength;
          RUN_vel(1,PAR_isAxis) = execVec(2,RUN_idx) / MvmtPerf;
          currStepTimeLength = currStepTimeLength * MvmtPerf;
        (default) -> Axis_X.Start_run.execute_movement.idle
        Axis_X.Start_run.execute_movement.idle -> Axis_X.Start_run.execute_movement.getOwnPerfCoeff [commented out] : after(currStepTimeLength * MvmtPerfEval_sendOwnVal,sec)
        Axis_X.Start_run.execute_movement.getOwnPerfCoeff -> Axis_X.Start_run.execute_movement.getMutualPerformance [commented out] : after(currStepTimeLength * (MvmtPerfEval_collectVal - MvmtPerfEval_sendOwnVal),sec)
      (default) -> Axis_X.Start_run.Send_command
      (junction 638) -> Axis_X.Start_run.Send_command [order 2]
      Axis_X.Start_run.Send_command -> Axis_X.Start_run.execute_movement
      Axis_X.Start_run.execute_movement -> (junction 638) : after(currStepTimeLength,sec)
    state DONE
      entry:
      send(axis_done);
    (default) -> Axis_X.Start_Idle
    Axis_X.Start_Idle -> Axis_X.Hermite_Interpolation
    Axis_X.Hermite_Interpolation -> Axis_X.Koordinationsvektor
    Axis_X.Koordinationsvektor -> Axis_X.Koordinationsvektor_austauschen
    Axis_X.Koordinationsvektor_austauschen -> Axis_X.Wait_for_cVectors [order 1] : [axisHasSentCVector == 1]
    Axis_X.Wait_for_cVectors -> Axis_X.Find_Consensus : [FLAG_cVectors_complete == 1]
    Axis_X.Find_Consensus -> Axis_X.Start_run : [FLAG_allAxesReady == 1]
    (junction 638) -> Axis_X.DONE [order 1] : [RUN_idx == RUN_num_steps]
  state Axis_Y [parallel]
    settings: executionOrder=3
    state Start_Idle
      entry:
      registerAxis.data = true;
      send(registerAxis)
    state Hermite_Interpolation
      entry:
      if FLAG_doAkima == 1
      iP = funcs.DS_hermIntp(setP,setP_dist);
      else
      iP = setP;
      end
    state Koordinationsvektor
      entry:
      cVector_init = funcs.DS_gen_Cvector_init...
      (iP,PAR_isAxis,PAR_maxVel);
    state Koordinationsvektor_austauschen
      during:
      if FLAG_canSend_cVector == 1
      cVector_exchange = cVector_init;
      FLAG_canSend_cVector = 0;
      send(cVector_sent);
      axisHasSentCVector = 1;
      end
      Axis_Y.Koordinationsvektor_austauschen -> Axis_Y.Koordinationsvektor_austauschen [order 1]
    state Wait_for_cVectors
    state Find_Consensus
      entry: execVec = funcs.DS_find_Consensus(iP,cVectors,...
      PAR_execIteratorStepSize,PAR_isAxis);
      send(axis_ready);
    state Start_run
      entry:
      RUN_idx = 0;
      RUN_startPos(1,PAR_isAxis) = setP(PAR_isAxis,1);
      RUN_num_steps = size(execVec,2);
      state Send_command
        entry:
        RUN_idx = RUN_idx + 1;
        currCVector = cVectors(:,RUN_idx)' ./ VelOverride';
        currCVal = max(currCVector);
        currOverrideAdaptationFactor = execVec(3,RUN_idx) / currCVal; %individueller neuer Override Faktor für diese Achse
        currStepTimeLength = execVec(3,RUN_idx) / currOverrideAdaptationFactor;
        RUN_pos(1,PAR_isAxis) = execVec(1,RUN_idx);
        RUN_vel(1,PAR_isAxis) = execVec(2,RUN_idx) * currOverrideAdaptationFactor;
        MvmtPerf_accumulatedLagTime = MvmtPerf_accumulatedLagTime + (currStepTimeLength - execVec(3,RUN_idx));
        RUN_time(1,PAR_isAxis) = execVec(4,RUN_idx) + MvmtPerf_accumulatedLagTime; %wird nicht benutzt
        RUN_maxVel(1,PAR_isAxis) = PAR_maxVel;
        RUN_MvmtPerfFeedback(1,PAR_isAxis) = 0; %wird zZt nicht benutzt
      state execute_movement
        state idle
          entry:
          MvmtPerfCoeff.data = -1;
          send(MvmtPerfCoeff);
        state getOwnPerfCoeff [commented out]
          entry:
          MvmtPerfCoeff.data = GET_perfIndicator(PAR_isAxis);
          send(MvmtPerfCoeff);
        state getMutualPerformance [commented out]
          entry:
          MvmtPerf_accumulatedLagTime = MvmtPerf_accumulatedLagTime + (MvmtPerf-1) * currStepTimeLength;
          RUN_MvmtPerfFeedback(1,PAR_isAxis) = (MvmtPerf-1) * currStepTimeLength;
          RUN_vel(1,PAR_isAxis) = execVec(2,RUN_idx) / MvmtPerf;
          currStepTimeLength = currStepTimeLength * MvmtPerf;
        (default) -> Axis_Y.Start_run.execute_movement.idle
        Axis_Y.Start_run.execute_movement.idle -> Axis_Y.Start_run.execute_movement.getOwnPerfCoeff [commented out] : after(currStepTimeLength * MvmtPerfEval_sendOwnVal,sec)
        Axis_Y.Start_run.execute_movement.getOwnPerfCoeff -> Axis_Y.Start_run.execute_movement.getMutualPerformance [commented out] : after(currStepTimeLength * (MvmtPerfEval_collectVal - MvmtPerfEval_sendOwnVal),sec)
      (default) -> Axis_Y.Start_run.Send_command
      (junction 1151) -> Axis_Y.Start_run.Send_command [order 2]
      Axis_Y.Start_run.Send_command -> Axis_Y.Start_run.execute_movement
      Axis_Y.Start_run.execute_movement -> (junction 1151) : after(currStepTimeLength,sec)
    state DONE
      entry:
      send(axis_done);
    (default) -> Axis_Y.Start_Idle
    Axis_Y.Start_Idle -> Axis_Y.Hermite_Interpolation
    Axis_Y.Hermite_Interpolation -> Axis_Y.Koordinationsvektor
    Axis_Y.Koordinationsvektor -> Axis_Y.Koordinationsvektor_austauschen
    Axis_Y.Koordinationsvektor_austauschen -> Axis_Y.Wait_for_cVectors [order 1] : [axisHasSentCVector == 1]
    Axis_Y.Wait_for_cVectors -> Axis_Y.Find_Consensus : [FLAG_cVectors_complete == 1]
    Axis_Y.Find_Consensus -> Axis_Y.Start_run : [FLAG_allAxesReady == 1]
    (junction 1151) -> Axis_Y.DONE [order 1] : [RUN_idx == RUN_num_steps]
  state Axis_Z [parallel]
    settings: executionOrder=4
    state Start_Idle
      entry:
      registerAxis.data = true;
      send(registerAxis)
    state Hermite_Interpolation
      entry:
      if FLAG_doAkima == 1
      iP = funcs.DS_hermIntp(setP,setP_dist);
      else
      iP = setP;
      end
    state Koordinationsvektor
      entry:
      cVector_init = funcs.DS_gen_Cvector_init...
      (iP,PAR_isAxis,PAR_maxVel);
    state Koordinationsvektor_austauschen
      during:
      if FLAG_canSend_cVector == 1
      cVector_exchange = cVector_init;
      FLAG_canSend_cVector = 0;
      send(cVector_sent);
      axisHasSentCVector = 1;
      end
      Axis_Z.Koordinationsvektor_austauschen -> Axis_Z.Koordinationsvektor_austauschen [order 1]
    state Wait_for_cVectors
    state Find_Consensus
      entry: execVec = funcs.DS_find_Consensus(iP,cVectors,...
      PAR_execIteratorStepSize,PAR_isAxis);
      send(axis_ready);
    state Start_run
      entry:
      RUN_idx = 0;
      RUN_startPos(1,PAR_isAxis) = setP(PAR_isAxis,1);
      RUN_num_steps = size(execVec,2);
      state Send_command
        entry:
        RUN_idx = RUN_idx + 1;
        currCVector = cVectors(:,RUN_idx)' ./ VelOverride';
        currCVal = max(currCVector);
        currOverrideAdaptationFactor = execVec(3,RUN_idx) / currCVal; %individueller neuer Override Faktor für diese Achse
        currStepTimeLength = execVec(3,RUN_idx) / currOverrideAdaptationFactor;
        RUN_pos(1,PAR_isAxis) = execVec(1,RUN_idx);
        RUN_vel(1,PAR_isAxis) = execVec(2,RUN_idx) * currOverrideAdaptationFactor;
        MvmtPerf_accumulatedLagTime = MvmtPerf_accumulatedLagTime + (currStepTimeLength - execVec(3,RUN_idx));
        RUN_time(1,PAR_isAxis) = execVec(4,RUN_idx) + MvmtPerf_accumulatedLagTime; %wird nicht benutzt
        RUN_maxVel(1,PAR_isAxis) = PAR_maxVel;
        RUN_MvmtPerfFeedback(1,PAR_isAxis) = 0; %wird zZt nicht benutzt
      state execute_movement
        state idle
          entry:
          MvmtPerfCoeff.data = -1;
          send(MvmtPerfCoeff);
        state getOwnPerfCoeff [commented out]
          entry:
          MvmtPerfCoeff.data = GET_perfIndicator(PAR_isAxis);
          send(MvmtPerfCoeff);
        state getMutualPerformance [commented out]
          entry:
          MvmtPerf_accumulatedLagTime = MvmtPerf_accumulatedLagTime + (MvmtPerf-1) * currStepTimeLength;
          RUN_MvmtPerfFeedback(1,PAR_isAxis) = (MvmtPerf-1) * currStepTimeLength;
          RUN_vel(1,PAR_isAxis) = execVec(2,RUN_idx) / MvmtPerf;
          currStepTimeLength = currStepTimeLength * MvmtPerf;
        (default) -> Axis_Z.Start_run.execute_movement.idle
        Axis_Z.Start_run.execute_movement.idle -> Axis_Z.Start_run.execute_movement.getOwnPerfCoeff [commented out] : after(currStepTimeLength * MvmtPerfEval_sendOwnVal,sec)
        Axis_Z.Start_run.execute_movement.getOwnPerfCoeff -> Axis_Z.Start_run.execute_movement.getMutualPerformance [commented out] : after(currStepTimeLength * (MvmtPerfEval_collectVal - MvmtPerfEval_sendOwnVal),sec)
      (default) -> Axis_Z.Start_run.Send_command
      (junction 1195) -> Axis_Z.Start_run.Send_command [order 2]
      Axis_Z.Start_run.Send_command -> Axis_Z.Start_run.execute_movement
      Axis_Z.Start_run.execute_movement -> (junction 1195) : after(currStepTimeLength,sec)
    state DONE
      entry:
      send(axis_done);
    (default) -> Axis_Z.Start_Idle
    Axis_Z.Start_Idle -> Axis_Z.Hermite_Interpolation
    Axis_Z.Hermite_Interpolation -> Axis_Z.Koordinationsvektor
    Axis_Z.Koordinationsvektor -> Axis_Z.Koordinationsvektor_austauschen
    Axis_Z.Koordinationsvektor_austauschen -> Axis_Z.Wait_for_cVectors [order 1] : [axisHasSentCVector == 1]
    Axis_Z.Wait_for_cVectors -> Axis_Z.Find_Consensus : [FLAG_cVectors_complete == 1]
    Axis_Z.Find_Consensus -> Axis_Z.Start_run : [FLAG_allAxesReady == 1]
    (junction 1195) -> Axis_Z.DONE [order 1] : [RUN_idx == RUN_num_steps]
  data: inp_data function_input; iPoints function_output; iP_dist function_input; inp_data function_input; whichAxis function_input; cV_init function_output; maxV function_input; iPoints function_input; cVec function_input; execVec function_output; iteratorStep function_input; whichAxis function_input; inp_data function_input; iPoints function_output; iP_dist function_input; num_registeredAxes local =0; num_collectedCVectors local =0; iP local size=[numAxes maxVectorLengths]; cVector_init local size=[1 maxVectorLengths]; PAR_isAxis constant double =1; PAR_maxVel constant double =10; axisHasSentCVector local =0; execVec local size=[4 maxVectorLengths] =1; RUN_idx local size=1 =0; currStepTimeLength local =0; RUN_num_steps local =0; MvmtPerf_accumulatedLagTime local =0; currCVector local size=[1 numAxes] =zeros(1,numAxes); currCVal local =0; currOverrideAdaptationFactor local =1; iP local size=[numAxes maxVectorLengths]; cVector_init local size=[1 maxVectorLengths]; PAR_isAxis constant double =2; PAR_maxVel constant double =5; axisHasSentCVector local =0; execVec local size=[4 maxVectorLengths] =1; RUN_idx local size=1 =0; currStepTimeLength local =0; RUN_num_steps local =0; MvmtPerf_accumulatedLagTime local =0; currCVector local size=[1 numAxes] =zeros(1,numAxes); currCVal local =0; currOverrideAdaptationFactor local =1; iP local size=[numAxes maxVectorLengths]; cVector_init local size=[1 maxVectorLengths]; PAR_isAxis constant double =3; PAR_maxVel constant double =2; axisHasSentCVector local =0; execVec local size=[4 maxVectorLengths] =1; RUN_idx local size=1 =0; currStepTimeLength local =0; RUN_num_steps local =0; MvmtPerf_accumulatedLagTime local =0; currCVector local size=[1 numAxes] =zeros(1,numAxes); currCVal local =0; currOverrideAdaptationFactor local =1; setP input; setP_dist input; registerAxis local; FLAG_canSend_cVector local =1; cVector_exchange local size=[1 maxVectorLengths]; cVector_sent local =1; cVectors local size=[numAxes maxVectorLengths] =0; FLAG_cVectors_complete local =0; PAR_execIteratorStepSize constant double =1; axis_ready local =0; num_readyAxes local =0; FLAG_allAxesReady local =0; FLAG_doAkima local =0; axis_done local =0; FLAG_stopSim output =0; num_doneAxes local =0; RUN_maxVel output size=[1 numAxes] =zeros(1,numAxes); RUN_pos output size=[1 numAxes] =zeros(1,numAxes); RUN_startPos output size=[1 numAxes] =zeros(1,numAxes); RUN_time output size=[1 numAxes] =zeros(1,numAxes); RUN_vel output size=[1 numAxes] =zeros(1,numAxes); MvmtPerfEval_sendOwnVal parameter; GET_perfIndicator data_store_memory; MvmtPerfCoeff local =1; MvmtPerf local =1; RUN_MvmtPerfFeedback output size=[1 numAxes] =zeros(1,numAxes); MvmtPerfEval_collectVal parameter; VelOverride data_store_memory
  function iPoints = DS_hermIntp(inp_data,iP_dist):
    | function iPoints = DS_hermIntp(inp_data,iP_dist)
    |  
    | 
    | euklid_abstand = vecnorm(diff(inp_data,1,2));
    | 
    | laufparam = cumsum(euklid_abstand);
    | laufparam = laufparam / max(laufparam);
    | laufparam = [0 laufparam];
    | 
    | 
    | anzahl_stuetzpunkte = 150;
    | anzahl_dim = size(inp_data,1);
    | iPoints = zeros(anzahl_dim,anzahl_stuetzpunkte);
    | 
    | for i=1:anzahl_dim
    |    
    |     iPoints(i,:) = pchip(laufparam,inp_data(i,:),linspace(0,1,anzahl_stuetzpunkte));
    |     
    | end
    | 
    | end
  function cV_init = DS_gen_Cvector_init(inp_data,whichAxis,maxV):
    | function cV_init = DS_gen_Cvector_init(inp_data,whichAxis,maxV)
    |  
    | safety_margin = 0.2; % max. Geschwindigkeit wird auf 80% der eigentlichen Fähigkeit der Achse festgelegt
    | 
    | wegdaten_raw = inp_data(whichAxis,:);
    | 
    | streckensegmente_raw = diff(wegdaten_raw);
    | 
    | 
    | zeitsegmente_raw = streckensegmente_raw ./ (maxV * (1 - safety_margin));
    | 
    | 
    | cV_init = abs(zeitsegmente_raw);
    | 
    | 
    | end
  function execVec = DS_find_Consensus(iPoints,cVec,iteratorStep,whichAxis):
    | function execVec = DS_find_Consensus(iPoints,cVec,iteratorStep,whichAxis)
    | 
    | cVector = max(cVec);
    | 
    | if(iteratorStep > 1)
    |    
    |     if(mod(size(iPoints,2)-1,iteratorStep) == 0)
    |         
    |         array_size = (size(iPoints,2) - 1) / iteratorStep;
    |         iPoints_relevant = zeros(1,array_size);
    |         
    |     else
    |        
    |         array_size = floor((size(iPoints,2) - 1) / iteratorStep) + 1;
    |         iPoints_relevant = zeros(1,array_size);
    |         
    |     end
    |     
    |     
    |     iPoints_relevant = iPoints(whichAxis,1:iteratorStep:end);
    |     
    |     % Neue Zeitabschnitte berechnen
    |     for ii=1:array_size-1
    |        
    |         currIdx = ((ii-1) * iteratorStep) + 1;
    |         zP = cVec(1,currIdx : currIdx + iteratorStep);
    |         
    |         zeitabschnitte = sum(zP);
    |         
    |     end
    | 
    |     
    | else
    |    
    |     iPoints_relevant = iPoints(whichAxis,:);
    | 
    |     
    | end
    | 
    |     wegabschnitte = diff(iPoints_relevant(1,:));
    |     zeitabschnitte = cVector;
    |     absolute_zeitpunkte = cumsum(zeitabschnitte);
    |     
    |     geschwindigkeiten = abs(wegabschnitte ./ zeitabschnitte);
    |     
    |     execVec = [iPoints_relevant(2:end);...
    |         geschwindigkeiten;...
    |         zeitabschnitte;...
    |         absolute_zeitpunkte];
    | 
    | 
    | 
    | end
  function iPoints = DS_hermIntp_old(inp_data,iP_dist):
    | function iPoints = DS_hermIntp_old(inp_data,iP_dist)
    |  
    | x = inp_data(1,:);
    | y = inp_data(2,:);
    | 
    | x_zwischenpunkte = (x(1):iP_dist:x(end));
    | 
    | y_interpoliert = pchip(x,y,x_zwischenpunkte);
    | 
    | iPoints = [x_zwischenpunkte; y_interpoliert];
    | 
    | 
    | end
